simulink model "sampleTime"  (R2017b)
settings: Solver=VariableStepAuto  StartTime=0.0  StopTime=3  RelTol=1e-3
settings Model: Creator=alic  LastModifiedBy=alic

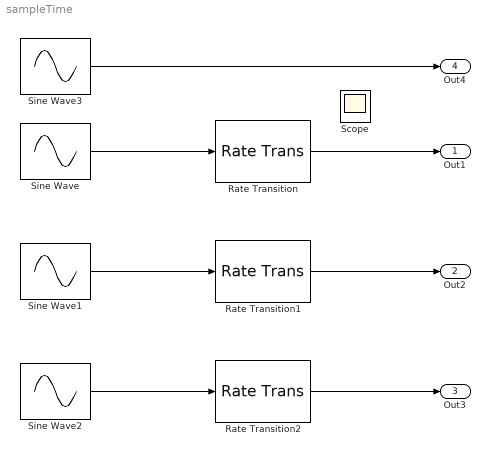
== system sampleTime ==
  Rate Transition : RateTransition  InitialCondition=0.5
  Rate Transition1 : RateTransition  InitialCondition=2
  Rate Transition2 : RateTransition  InitialCondition=0.5
  Scope : Scope
  Sine Wave : Sin  Bias=1  SampleTime=0.1
  Sine Wave1 : Sin  Bias=1  SampleTime=0.2
  Sine Wave2 : Sin  Bias=1  SampleTime=0.3
  Sine Wave3 : Sin  Bias=1  SampleTime=0.2
  Out1 : Outport  SampleTime=0.2
  Out2 : Outport  Port=2  SampleTime=0.1
  Out3 : Outport  Port=3  SampleTime=0.3
  Out4 : Outport  Port=4  SampleTime=0.1
  wires:
  Rate Transition/1 -> Out1/1
  Rate Transition1/1 -> Out2/1
  Rate Transition2/1 -> Out3/1
  Sine Wave2/1 -> Rate Transition2/1
  Sine Wave1/1 -> Rate Transition1/1
  Sine Wave/1 -> Rate Transition/1
  Sine Wave3/1 -> Out4/1
